simulink model "modeldrone"  (R2015a)
settings: Solver=ode45  StartTime=0.0  StopTime=40  RelTol=1e-3
values from neighbouring files (symbols this model uses):
  b = 0.00004    (= 4e-05)    [Parametres.m]    (also in lissajou_curves_3D.m = 4)
  d = 0.000007    (= 7e-06)    [Parametres.m]
  Ix = 0.005    [Parametres.m]
  Iy = Ix    (= 0.005)    [Parametres.m]
  Iz = 0.01    [Parametres.m]
  Jr = 0.00005    (= 5e-05)    [Parametres.m]
  l = 0.25    [Parametres.m]
undefined symbols (not defined in the file or in its folder): m
libraries: simulink x1
settings Model: Creator=Oussama  LastModifiedBy=Oussama
settings SimscapeCC: SimscapeLogType=all  SimscapeLogDataHistory=10000

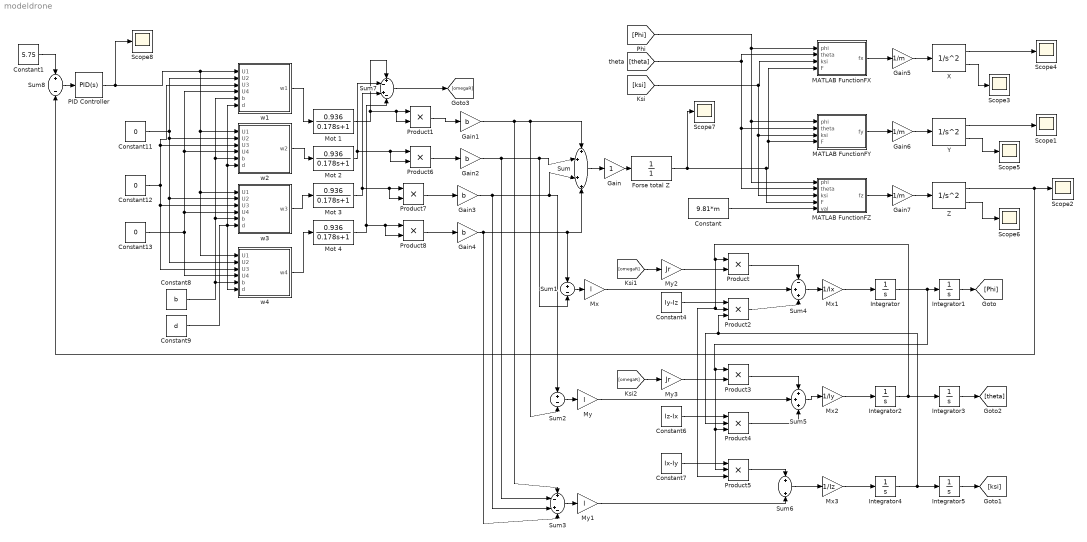
== system modeldrone ==
  Constant : Constant  Value=9.81*m
  Constant1 : Constant  Value=5.75
  Constant11 : Constant  Value=0
  Constant12 : Constant  Value=0
  Constant13 : Constant  Value=0
  Constant4 : Constant  Value=Iy-Iz
  Constant6 : Constant  Value=Iz-Ix
  Constant7 : Constant  Value=Ix-Iy
  Constant8 : Constant  Value=b
  Constant9 : Constant  Value=d
  Forse total Z : TransferFcn  Denominator=[0 1]
  Gain : Gain
  Gain{1..4} (4 alike) : Gain  Gain=b
  Gain5 : Gain  Gain=1/m
  Gain6 : Gain  Gain=1/m
  Gain7 : Gain  Gain=1/m
  Integrator{,1..5} (6 alike) : Integrator
  MATLAB FunctionFX : MATLAB Function  TreatAsAtomicUnit=on
  "MATLAB FunctionFY " : MATLAB Function  TreatAsAtomicUnit=on
  "MATLAB FunctionFZ " : MATLAB Function  TreatAsAtomicUnit=on
  Mot {1..4} (4 alike) : TransferFcn  Numerator=[0.936]  Denominator=[0.178 1]
  Mx : Gain  Gain=l
  Mx1 : Gain  Gain=1/Ix
  Mx2 : Gain  Gain=1/Iy
  Mx3 : Gain  Gain=1/Iz
  My : Gain  Gain=l
  My1 : Gain  Gain=l
  My2 : Gain  Gain=Jr
  My3 : Gain  Gain=Jr
  PID Controller : simulink/Continuous/PID Controller  Controller=PID  TimeDomain=Continuous-time  SampleTime=-1  IntegratorMethod=Forward Euler  FilterMethod=Forward Euler  Form=Parallel  UseFilter=on  ControllerParametersSource=internal  P=15  I=0.1  D=0.6  N=100  InitialConditionSource=internal  InitialConditionForIntegrator=0  InitialConditionForFilter=0  ExternalReset=none  LimitOutput=off  UpperSaturationLimit=inf  LowerSaturationLimit=-inf  LinearizeAsGain=on  AntiWindupMode=none  Kb=1  TrackingMode=off  Kt=1  PParamMin=[]  PParamMax=[]  IParamMin=[]  IParamMax=[]  DParamMin=[]  DParamMax=[]  NParamMin=[]  NParamMax=[]  KbParamMin=[]  KbParamMax=[]  KtParamMin=[]  KtParamMax=[]  POutMin=[]  POutMax=[]  IOutMin=[]  IOutMax=[]  DOutMin=[]  DOutMax=[]  NOutMin=[]  NOutMax=[]  KbOutMin=[]  KbOutMax=[]  KtOutMin=[]  KtOutMax=[]  IntegratorOutMin=[]  IntegratorOutMax=[]  FilterOutMin=[]  FilterOutMax=[]  SumOutMin=[]  SumOutMax=[]  SumI1OutMin=[]  SumI1OutMax=[]  SumI2OutMin=[]  SumI2OutMax=[]  SumI3OutMin=[]  SumI3OutMax=[]  SumDOutMin=[]  SumDOutMax=[]  SaturationOutMin=[]  SaturationOutMax=[]  IntegratorContinuousStateAttributes=''  IntegratorStateMustResolveToSignalObject=off  IntegratorRTWStateStorageClass=Auto  FilterContinuousStateAttributes=''  FilterStateMustResolveToSignalObject=off  FilterRTWStateStorageClass=Auto  DifferentiatorICPrevScaledInput=0  DifferentiatorOutMin=[]  DifferentiatorOutMax=[]
  Product{,1,3,6..8} (6 alike) : Product
  Product2 : Product  Inputs=3
  Product4 : Product  Inputs=3
  Product5 : Product  Inputs=3
  Scope{1..8} (8 alike) : Scope
      Scope3 settings: SaveName=ScopeData2
      Scope4 settings: SaveName=ScopeData3
      Scope5 settings: SaveName=ScopeData4
      Scope6 settings: SaveName=ScopeData5
      Scope7 settings: SaveName=ScopeData6
      Scope8 settings: SaveName=ScopeData7
  Sum : Sum  Inputs=++++
  Sum1 : Sum  Inputs=+-
  Sum2 : Sum  Inputs=+-
  Sum3 : Sum  Inputs=+-+-
  Sum4 : Sum  Inputs=-++
  Sum5 : Sum  Inputs=+++
  Sum6 : Sum
  Sum7 : Sum  Inputs=+-+-
  Sum8 : Sum  Inputs=+-
  X : SecondOrderIntegrator
  Y : SecondOrderIntegrator
  Z : SecondOrderIntegrator
  "w1 " : MATLAB Function  TreatAsAtomicUnit=on
  w2 : MATLAB Function  TreatAsAtomicUnit=on
  w3 : MATLAB Function  TreatAsAtomicUnit=on
  w4 : MATLAB Function  TreatAsAtomicUnit=on
  wires:
  Mot 2/1 -> Product6/2, Product6/1, Sum7/2
  Mot 3/1 -> Product7/2, Product7/1, Sum7/3
  Mot 4/1 -> Product8/2, Product8/1, Sum7/4
  Mot 1/1 -> Product1/2, Product1/1, Sum7/1
  Sum/1 -> Gain/1
  Gain/1 -> Forse total Z/1
  Gain4/1 -> Sum3/4, Sum1/1, Sum/4
  Sum1/1 -> Mx/1
  Gain2/1 -> Sum3/2, Sum/2, Sum1/2
  Gain3/1 -> Sum3/3, Sum2/1, Sum/3
  Sum2/1 -> My/1
  Gain1/1 -> Sum/1, Sum2/2, Sum3/1
  Sum3/1 -> My1/1
  Forse total Z/1 -> Scope7/1, "MATLAB FunctionFZ "/4(F), "MATLAB FunctionFY "/4(F), MATLAB FunctionFX/4(F)
  [Phi] -> MATLAB FunctionFX/1(phi), "MATLAB FunctionFY "/1(phi), "MATLAB FunctionFZ "/1(phi)
  [theta] -> "MATLAB FunctionFZ "/2(theta), "MATLAB FunctionFY "/2(theta), MATLAB FunctionFX/2(theta)
  [ksi] -> "MATLAB FunctionFZ "/3(ksi), "MATLAB FunctionFY "/3(ksi), MATLAB FunctionFX/3(ksi)
  Gain5/1 -> X/1
  MATLAB FunctionFX/1(fx) -> Gain5/1
  Gain6/1 -> Y/1
  "MATLAB FunctionFY "/1(fy) -> Gain6/1
  Gain7/1 -> Z/1
  "MATLAB FunctionFZ "/1(fz) -> Gain7/1
  Constant/1 -> "MATLAB FunctionFZ "/5(val)
  w3/1(w3) -> Mot 3/1
  w4/1(w4) -> Mot 4/1
  w2/1(w2) -> Mot 2/1
  "w1 "/1(w1) -> Mot 1/1
  Product/1 -> Sum4/1
  Mx/1 -> Sum4/2
  Sum4/1 -> Mx1/1
  Product2/1 -> Sum4/3
  Constant4/1 -> Product2/1
  Mx1/1 -> Integrator/1
  My2/1 -> Product/2
  Sum5/1 -> Mx2/1
  Mx2/1 -> Integrator2/1
  Sum6/1 -> Mx3/1
  Mx3/1 -> Integrator4/1
  Integrator4/1 -> Product4/2, Product2/3, Integrator5/1
  Integrator3/1 -> [theta]
  Integrator5/1 -> [ksi]
  Integrator1/1 -> [Phi]
  My3/1 -> Product3/2
  Integrator/1 -> Product5/2, Product4/3, Product3/1, Integrator1/1
  Product3/1 -> Sum5/1
  My/1 -> Sum5/2
  Constant6/1 -> Product4/1
  Constant7/1 -> Product5/1
  Integrator2/1 -> Product5/3, Product2/2, Product/1, Integrator3/1
  Product5/1 -> Sum6/1
  My1/1 -> Sum6/2
  Constant8/1 -> "w1 "/5(b), w2/5(b), w3/5(b), w4/5(b)
  Constant9/1 -> w4/6(d), w2/6(d), "w1 "/6(d), w3/6(d)
  Product4/1 -> Sum5/3
  Sum8/1 -> PID Controller/1
  Constant11/1 -> w2/2(U2), w3/2(U2), w4/2(U2), "w1 "/2(U2)
  Constant12/1 -> w3/3(U3), w4/3(U3), w2/3(U3), "w1 "/3(U3)
  Constant13/1 -> w4/4(U4), "w1 "/4(U4), w2/4(U4), w3/4(U4)
  Sum7/1 -> [omegaR]
  [omegaR] -> My2/1
  [omegaR] -> My3/1
  X/1 -> Scope4/1
  Y/1 -> Scope1/1
  X/2 -> Scope3/1
  Y/2 -> Scope5/1
  Z/2 -> Scope6/1
  Product1/1 -> Gain1/1
  Product6/1 -> Gain2/1
  Product7/1 -> Gain3/1
  Product8/1 -> Gain4/1
  Z/1 -> Sum8/2, Scope2/1
  PID Controller/1 -> Scope8/1, w4/1(U1), w3/1(U1), w2/1(U1), "w1 "/1(U1)
  Constant1/1 -> Sum8/1

== matlab function modeldrone/MATLAB FunctionFY  ==
  data: phi input; fy output; theta input; ksi input; F input
function fy = fcn(phi, theta, ksi, F)
%#codegen

fy = (cos(phi)*sin(theta)*sin(ksi)+sin(phi)*cos(ksi))*F;

== matlab function modeldrone/MATLAB FunctionFX ==
  data: phi input; fx output; theta input; ksi input; F input
function fx = fcn(phi, theta, ksi, F)
%#codegen

fx = (cos(phi)*sin(theta)*cos(ksi)+sin(phi)*sin(ksi))*F;

== matlab function modeldrone/MATLAB FunctionFZ  ==
  data: phi input; fz output; theta input; ksi input; F input; val input
function fz = fcn(phi, theta, ksi, F, val)
%#codegen

fz = (cos(phi)*cos(theta))*F-val;

== matlab function modeldrone/w1  ==
  data: U1 input; w1 output; U2 input; U3 input; U4 input; b input; d input
function w1 = fcn(U1, U2, U3, U4,b,d)
%#codegen

w1 = sqrt(0.25/b*U1-0.5/b*U3+0.25/d*U4)+U2-U2;

== matlab function modeldrone/w2 ==
  data: U1 input; w2 output; U2 input; U3 input; U4 input; b input; d input
function w2 = fcn(U1, U2, U3, U4,b,d)
%#codegen

w2 = sqrt(0.25/b*U1-0.5/b*U2-0.25/d*U4)+U3-U3;

== matlab function modeldrone/w3 ==
  data: U1 input; w3 output; U2 input; U3 input; U4 input; b input; d input
function w3 = fcn(U1, U2, U3, U4,b,d)
%#codegen

w3 = sqrt(0.25/b*U1+0.5/b*U3+0.25/d*U4);

== matlab function modeldrone/w4 ==
  data: U1 input; w4 output; U2 input; U3 input; U4 input; b input; d input
function w4 = fcn(U1, U2, U3, U4,b,d)
%#codegen

w4 = sqrt(0.25/b*U1+0.5/b*U2-0.25/d*U4);
